simulink model "SCARA_Ass4_Arm_Control_2009"  (Simulink 7.4)
settings: Solver=FixedStepDiscrete  StartTime=0.0  StopTime=inf  FixedStep=0.00001  RelTol=1e-3
undefined symbols (not defined in the file): DiscIntNeverNeededParam
libraries: vrlib x6, dspmtrx3 x5, simulink x2, RT x1, dspinverses x1
settings Model: Creator=Mengchen  LastModifiedBy=t6z8
settings OptimizationCC: ExpressionDepthLimit=128  InitFltsAndDblsToZero=on
settings DebuggingCC: AlgebraicLoopMsg=error  SaveWithParameterizedLinksMsg=none  StateNameClashWarn=none  StrictBusMsg=ErrorLevel1
settings HardwareCC: TargetEndianess=LittleEndian  TargetHWDeviceType=MATLAB Host
settings RTWCC: ProcessScript=grt_make_rtw_hook  CustomHeaderCode="#include \"haptics.h\""  CustomInclude="\"C:\\Program Files\\novint\\HDAL_SDK_1.1.0_Beta\\include\""  TargetLang=C++
settings CodeAppCC: CustomSymbolStrType=$N$R$M_T

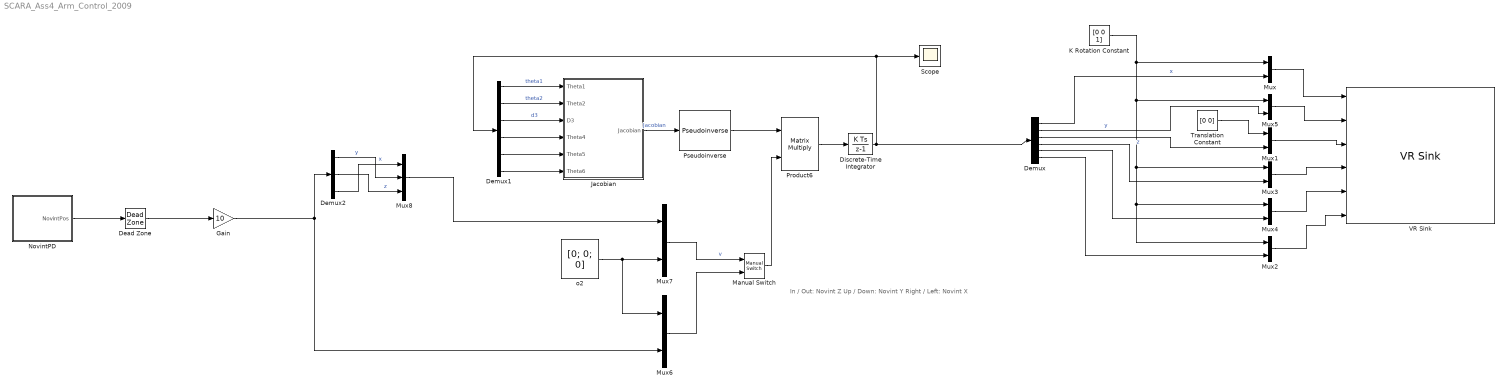
== system SCARA_Ass4_Arm_Control_2009 ==
  note: In / Out: Novint Z
      | Up / Down: Novint Y
      | Right / Left: Novint X
  Dead Zone : DeadZone  SaturateOnIntegerOverflow=on
  Demux : Demux  Outputs=6
  Demux1 : Demux  Outputs=6
  Demux2 : Demux  Outputs=3
  Discrete-Time Integrator : DiscreteIntegrator  InitialCondition=[0; -pi/2; 0; 0; 0; 0]  SampleTime=0.001  OutDataType=fixdt(1, 16)  OutScaling=2^0  ICPrevOutput=DiscIntNeverNeededParam  ICPrevScaledInput=DiscIntNeverNeededParam
  Gain : Gain  Gain=10  ParameterDataType=fixdt(1, 16)  ParameterScaling=2^0  OutDataType=fixdt(1, 16)  OutScaling=2^0
  Jacobian : Subsystem
  K Rotation Constant : Constant  Value=[0 0 1]
  Manual Switch : simulink/Signal Routing/Manual Switch  SystemSampleTime=-1  sw=0  action=0  varsize=off
  Mux{,1..7} (8 alike) : Mux  Inputs=2
  Mux8 : Mux  Inputs=3
  NovintPD : Subsystem
  Product6 : Product  Multiplication=Matrix(*)  OutDataType=fixdt(1, 16)  OutScaling=2^0  RndMeth=Zero
  Pseudoinverse : dspinverses/Pseudoinverse  wanterr=off
  Scope : Scope
      settings: SaveName=ScopeData3
  Translation Constant : Constant  Value=[0 0]
  VR Sink : vrlib/VR Sink  InstantiateOnLoad=on  SampleTime=-1  ViewEnable=on  RemoteChange=off  RemoteView=on  FieldsWritten=Link_0_Rotation.rotation.4.1.double#Link_1_Rotation.rotation.4.1.double#Link_2_Translation.translation.3.1.double#Link_3_Rotation.rotation.4.1.double#Link_4_Rotation.rotation.4.1.double#Link_5_Rotation.rotation.4.1.double  WorldFileName=SCARAWORLD.WRL  AutoView=off  VideoDimensions=[]
  o2 : Constant  Value=[0; 0; 0]  VectorParams1D=off  OutDataType=fixdt(1, 16)  OutScaling=2^0
  wires:
  K Rotation Constant/1 -> Mux/1, Mux3/1, Mux4/1, Mux2/1, Mux5/1
  Mux/1 -> VR Sink/1
  Mux1/1 -> VR Sink/3
  Translation Constant/1 -> Mux1/1
  Mux3/1 -> VR Sink/4
  Mux4/1 -> VR Sink/5
  Mux2/1 -> VR Sink/6
  Mux5/1 -> VR Sink/2
  Demux/1 -> Mux/2  "x"
  o2/1 -> Mux7/2, Mux6/1
  Pseudoinverse/1 -> Product6/1
  Product6/1 -> Discrete-Time Integrator/1
  Demux2/1 -> Mux8/2  "y"
  Demux2/2 -> Mux8/3  "z"
  Mux8/1 -> Mux7/1
  Demux/2 -> Mux5/2  "y"
  Demux/3 -> Mux1/2  "z"
  Demux2/3 -> Mux8/1  "x"
  Dead Zone/1 -> Gain/1
  Demux1/1 -> Jacobian/1(Theta1)  "theta1"
  Demux1/2 -> Jacobian/2(Theta2)  "theta2"
  Demux1/3 -> Jacobian/3(D3)  "d3"
  Jacobian/1(Jacobian) -> Pseudoinverse/1  "Jacobian"
  Discrete-Time Integrator/1 -> Demux/1, Demux1/1, Scope/1
  Demux1/4 -> Jacobian/4(Theta4)
  Demux1/5 -> Jacobian/5(Theta5)
  Demux1/6 -> Jacobian/6(Theta6)
  Gain/1 -> Demux2/1, Mux6/2
  NovintPD/1(NovintPos) -> Dead Zone/1
  Demux/4 -> Mux3/2
  Demux/5 -> Mux4/2
  Demux/6 -> Mux2/2
  Manual Switch/1 -> Product6/2
  Mux7/1 -> Manual Switch/1  "v"
  Mux6/1 -> Manual Switch/2

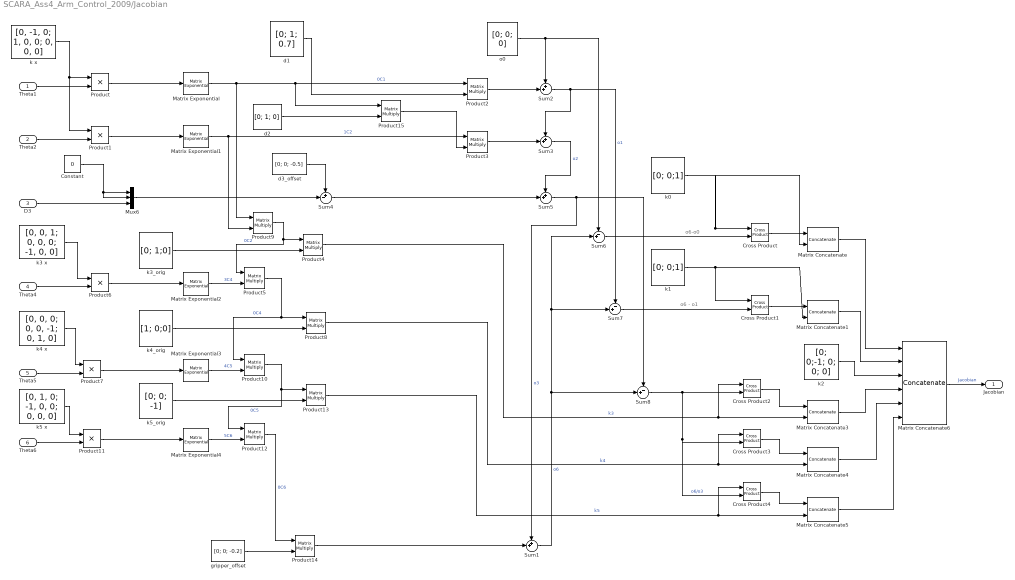
== system SCARA_Ass4_Arm_Control_2009/Jacobian ==
  note: o6 - o1
  note: o6-o0
  Theta1 : Inport
  Theta2 : Inport  Port=2
  D3 : Inport  Port=3
  Theta4 : Inport  Port=4
  Theta5 : Inport  Port=5
  Theta6 : Inport  Port=6
  Constant : Constant  Value=0  OutDataType=fixdt(1, 16)  OutScaling=2^0
  Cross Product{,1..4} (5 alike) : vrlib/Utilities/Cross Product  SystemSampleTime=-1
  Matrix Concatenate{,1,3..5} (5 alike) : Concatenate  Mode=Multidimensional array
  Matrix Concatenate6 : Concatenate  NumInputs=6  Mode=Multidimensional array  ConcatenateDimension=2
  Matrix Exponential{,1..4} (5 alike) : dspmtrx3/Matrix Exponential  SystemSampleTime=-1
  Mux6 : Mux  Inputs=3
  Product{,1,6..7,11} (5 alike) : Product  OutDataType=fixdt(1, 16)  OutScaling=2^0  RndMeth=Zero
  Product{2..5,8..10,12..15} (11 alike) : Product  Multiplication=Matrix(*)  OutDataType=fixdt(1, 16)  OutScaling=2^0  RndMeth=Zero
  Sum{1..3,5} (4 alike) : Sum  Inputs=++|
  Sum4 : Sum  Inputs=+-|
  Sum6 : Sum  Inputs=-+|
  Sum7 : Sum  Inputs=-+|
  Sum8 : Sum  Inputs=-+|
  d1 : Constant  Value=[0; 1; 0.7]  VectorParams1D=off  OutDataType=fixdt(1, 16)  OutScaling=2^0
  d2 : Constant  Value=[0; 1; 0]  VectorParams1D=off  OutDataType=fixdt(1, 16)  OutScaling=2^0
  d3_offset : Constant  Value=[0; 0; -0.5]  VectorParams1D=off  OutDataType=fixdt(1, 16)  OutScaling=2^0
  gripper_offset : Constant  Value=[0; 0; -0.2]  VectorParams1D=off  OutDataType=fixdt(1, 16)  OutScaling=2^0
  k x : Constant  Value=[0, -1, 0; 1, 0, 0; 0, 0, 0]  VectorParams1D=off  OutDataType=fixdt(1, 16)  OutScaling=2^0
  k0 : Constant  Value=[0; 0;1]  VectorParams1D=off  OutDataType=fixdt(1, 16)  OutScaling=2^0
  k1 : Constant  Value=[0; 0;1]  VectorParams1D=off  OutDataType=fixdt(1, 16)  OutScaling=2^0
  k2 : Constant  Value=[0; 0;-1; 0; 0; 0]  VectorParams1D=off  OutDataType=fixdt(1, 16)  OutScaling=2^0
  k3 x : Constant  Value=[0, 0, 1; 0, 0, 0; -1, 0, 0]  VectorParams1D=off  OutDataType=fixdt(1, 16)  OutScaling=2^0
  k3_orig : Constant  Value=[0; 1;0]  VectorParams1D=off  OutDataType=fixdt(1, 16)  OutScaling=2^0
  k4 x : Constant  Value=[0, 0, 0; 0, 0, -1; 0, 1, 0]  VectorParams1D=off  OutDataType=fixdt(1, 16)  OutScaling=2^0
  k4_orig : Constant  Value=[1; 0;0]  VectorParams1D=off  OutDataType=fixdt(1, 16)  OutScaling=2^0
  k5 x : Constant  Value=[0, 1, 0; -1, 0, 0; 0, 0, 0]  VectorParams1D=off  OutDataType=fixdt(1, 16)  OutScaling=2^0
  k5_orig : Constant  Value=[0; 0; -1]  VectorParams1D=off  OutDataType=fixdt(1, 16)  OutScaling=2^0
  o0 : Constant  Value=[0; 0; 0]  VectorParams1D=off  OutDataType=fixdt(1, 16)  OutScaling=2^0
  Jacobian : Outport
  wires:
  Matrix Concatenate3/1 -> Matrix Concatenate6/4
  Matrix Concatenate4/1 -> Matrix Concatenate6/5
  Matrix Concatenate5/1 -> Matrix Concatenate6/6
  Sum4/1 -> Sum5/2
  Sum5/1 -> Sum1/1, Sum8/1  "o3"
  Sum6/1 -> Cross Product/2
  k0/1 -> Matrix Concatenate/2, Cross Product/1
  Cross Product/1 -> Matrix Concatenate/1
  Sum7/1 -> Cross Product1/2
  Cross Product1/1 -> Matrix Concatenate1/1
  k1/1 -> Matrix Concatenate1/2, Cross Product1/1
  Matrix Concatenate/1 -> Matrix Concatenate6/1
  Matrix Concatenate1/1 -> Matrix Concatenate6/2
  Matrix Exponential/1 -> Product2/1, Product15/1, Product9/1  "0C1"
  Matrix Exponential1/1 -> Product3/1, Product9/2  "1C2"
  d1/1 -> Product2/2
  o0/1 -> Sum2/1, Sum6/1
  Product2/1 -> Sum2/2
  Sum2/1 -> Sum3/1, Sum7/1  "o1"
  Product3/1 -> Sum3/2
  Sum3/1 -> Sum5/1  "o2"
  d3_offset/1 -> Sum4/1
  k x/1 -> Product/1, Product1/1
  Product/1 -> Matrix Exponential/1
  Product1/1 -> Matrix Exponential1/1
  Constant/1 -> Mux6/1, Mux6/2
  Mux6/1 -> Sum4/2
  Theta1/1 -> Product/2
  Theta2/1 -> Product1/2
  D3/1 -> Mux6/3
  Matrix Concatenate6/1 -> Jacobian/1  "Jacobian"
  k3_orig/1 -> Product4/2
  Product4/1 -> Matrix Concatenate3/2, Cross Product2/1  "k3"
  Theta4/1 -> Product6/2
  k3 x/1 -> Product6/1
  Product6/1 -> Matrix Exponential2/1
  k4 x/1 -> Product7/1
  Theta5/1 -> Product7/2
  Product7/1 -> Matrix Exponential3/1
  Product9/1 -> Product4/1, Product5/1  "0C2"
  Product5/1 -> Product8/1, Product10/1  "0C4"
  k4_orig/1 -> Product8/2
  Product8/1 -> Matrix Concatenate4/2, Cross Product3/1  "k4"
  Theta6/1 -> Product11/2
  k5 x/1 -> Product11/1
  Product11/1 -> Matrix Exponential4/1
  Matrix Exponential4/1 -> Product12/2  "5C6"
  Product10/1 -> Product12/1, Product13/1  "0C5"
  k5_orig/1 -> Product13/2
  Product13/1 -> Matrix Concatenate5/2, Cross Product4/1  "k5"
  gripper_offset/1 -> Product14/2
  Product12/1 -> Product14/1  "0C6"
  Product14/1 -> Sum1/2
  k2/1 -> Matrix Concatenate6/3
  Sum1/1 -> Sum6/2, Sum7/2, Sum8/2  "o6"
  Cross Product2/1 -> Matrix Concatenate3/1
  Sum8/1 -> Cross Product2/2, Cross Product3/2, Cross Product4/2  "o6/o3"
  Cross Product3/1 -> Matrix Concatenate4/1
  Cross Product4/1 -> Matrix Concatenate5/1
  d2/1 -> Product15/2
  Product15/1 -> Product3/2
  Matrix Exponential2/1 -> Product5/2  "3C4"
  Matrix Exponential3/1 -> Product10/2  "4C5"

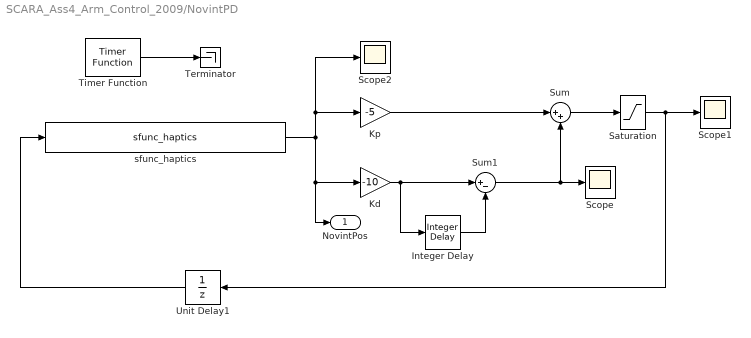
== system SCARA_Ass4_Arm_Control_2009/NovintPD ==
  Integer Delay : simulink/Discrete/Integer Delay  vinit=0.0  samptime=-1  NumDelays=2
  Kd : Gain  Gain=-10
  Kp : Gain  Gain=-5
  Saturation : Saturate  UpperLimit=200  LowerLimit=-200
  Scope : Scope
      settings: YMin=-0.9  YMax=0.6
  Scope1 : Scope
  Scope2 : Scope
      settings: YMin=-1.2  YMax=1  SaveName=ScopeData2
  Sum : Sum  Inputs=|++
  Sum1 : Sum  Inputs=|+-
  Terminator : Terminator
  Timer Function : RT/Timer Function  step1=0.9  priority1=HIGH  ThPriority1=TIME CRITICAL
  Unit Delay1 : UnitDelay  SampleTime=-1
  sfunc_haptics : S-Function  FunctionName=sfunc_haptics  EnableBusSupport=off  mask(Legacy Function){SFunctionSpec=void falconPlant(double u1[3], double y1[3]), ShowSpec=on}
      mask prompts: ShowSpec "Display function specification"
      mask help:
      | This block allows you to call the legacy functions specified by the following Legacy Code Tool definition:
      | def.SFunctionName = 'sfunc_haptics';
      | def.OutputFcnSpec = 'void falconPlant(double u1[3], double y1[3])';
      | def.StartFcnSpec = 'createHaptics()';
      | def.TerminateFcnSpec = 'deleteHaptics()';
      | def.HeaderFiles = {'haptics.h'};
      | def.SourceFiles = {'haptics.cpp'};
      | def.HostLibFiles = {'hdl.lib'};
      | def.TargetLibFiles = {'hdl.lib'};
      | def.IncPaths = {'C:\Program Files (x86)\novint\HDAL_SDK_2.1.3\include'};
      | def.LibPaths = {'C:\Program Files (x86)\novint\HDAL_SDK_2.1.3\lib'};
      | def.Options.useTlcWithAccel = false;
      | def.Options.language = 'C++';
      mask Help: <p>This block was generated automatically by the Legacy Code Tool. For detailed help on this tool, call<a href="matlab:legacy_code('help')"> legacy_code('help')</a>.</p>
      mask CallbackString:
      | |if strcmp(get_param(gcbh, 'ShowSpec'), 'on')
      |   set_param(gcbh, 'MaskDisplay', sprintf('fprintf(''%s'');', get_param(gcbh, 'SFunctionSpec')));
      | else
      |   set_param(gcbh, 'MaskDisplay', sprintf('fprintf(''%s'');', get_param(gcbh, 'FunctionName')));
      | end
      mask Display: fprintf('void falconPlant(double u1[3], double y1[3])');
  NovintPos : Outport
  wires:
  Saturation/1 -> Scope1/1, Unit Delay1/1
  Sum/1 -> Saturation/1
  Kp/1 -> Sum/1
  Sum1/1 -> Sum/2, Scope/1
  Integer Delay/1 -> Sum1/2
  Kd/1 -> Sum1/1, Integer Delay/1
  Unit Delay1/1 -> sfunc_haptics/1
  sfunc_haptics/1 -> Kp/1, Scope2/1, NovintPos/1, Kd/1
  Timer Function/1 -> Terminator/1
